simulink library "vmc"  (R2021b)
settings: Solver=VariableStepAuto  StartTime=0.0  StopTime=10.0  RelTol=1e-3
undefined symbols (not defined in the file or in its folder): AVMC_ACCDeltaTqIGain_X_kph, AVMC_ACCDeltaTqIGain_Y_mps2, AVMC_ACCDeltaTqPGain_X_kph, AVMC_ACCDeltaTqPGain_Y_kph, AVMC_ACCLongSteadyCtrl_X_kph, AVMC_AggressJerkPCT4AT_X_kph, AVMC_AggressJerkPCT_X_kph, AVMC_AggressLimitPCT4AT_X_kph, AVMC_AggressLimitPCT_X_kph, AVMC_CCLongSteadyCtrl_X_kph, AVMC_DISCDeltaTqIGain_X_kph, AVMC_DISCDeltaTqIGain_Y_mps2, AVMC_DISCDeltaTqPGain_X_kph, AVMC_DISCDeltaTqPGain_Y_kph, AVMC_DISCTrunAccJerk_X_s, AVMC_DISCTrunAccLimit_X_s, AVMC_ESCRegenOut_X_kph, AVMC_ESCRegenOut_Y_Deg, AVMC_ESCRegenOutEnSpd_X_Deg, AVMC_ISOAccLimit_X_mps, AVMC_ISODecLimit_X_mps, AVMC_ISOJerk_X_mps, AVMC_LatESCRegenOut_X_kph, AVMC_LatESCRegenOut_Y_Deg, AVMC_LongAccDeadZone_X_kph, AVMC_LongAccFiltTsforP2_X_Gps, AVMC_MCPresBaseTq_X_bar, AVMC_MSALongSteadyCtrl_X_kph, AVMC_MSAPedalOvrd2_X_kph, AVMC_MSAPedalOvrd_X_kph, AVMC_MSASpdBand_X_kph, AVMC_MSATqDownEndTq_X_kph, AVMC_MSATqDownTime_X_kph, AVMC_OPDDisSlideRate_X_Deg, AVMC_RDCDetectTime_X_kph, AVMC_RDCDetectTime_Y_pct, AVMC_RDCEnSlideRate_X_Deg, AVMC_RearWhlTqRatio_X_Nm, AVMC_RearWhlTqRatio_Y_gps, AVMC_RearWhlTqSlipGain_X_rat, AVMC_RearWhlTqSlipGain_Y_kph, AVMC_RearWhlTqSTRGGain_X_deg, AVMC_RearWhlTqSTRGGain_Y_kph, AVMC_RWSRrTSA2RWSPos_X_deg, AVMC_RWSSAS2FrtTSA_X_deg, AVMC_RWSVehSPD2RWSCoef_X_kph, AVMC_SoftJerkPCT_X_kph, AVMC_SoftLimitPCT_X_kph, AVMC_StESCYaw_X_kph, AVMC_StESCYaw_Y_Deg, AVMC_StESCYawCom_X_kph, AVMC_StESCYawCom_Y_Gps, AVMC_TMSpdBaseTq_X_rpm, AVMC_VehHoldBDecMap_X_kph, AVMC_VehHoldDecCtrlTime_X_kph, AVMC_VehHoldMCPPass_X_deg, C_TASK_10MS_S, C_TASK_5MS_S, DEG2RAD, ENUM_ACCAVAIL_AVAILABLE ... (+409)
libraries: hcu_lib x74, simulink x68, simulink_extras x3, $bdroot x2
(part 13 of 15)

== system vmc/VMC/VMC/Slide Rate  Calculation/4Wheel Calculation/RR Wheel ==
  VVMC_4WheelLongAcc_Gps : Inport
  task_time_s : Inport  Port=2
  VINP_RRRawWhlSpeed_kph : Inport  Port=3
  VTQD_GearActualPosn_enum : Inport  Port=4
  AND4 : Logic  Inputs=3  AllPortsSameDT=off  OutDataTypeStr=boolean
  Abs3 : Abs
  Add : Sum
  Add{3,8,15..16} (4 alike) : Sum  Inputs=+-
  Constant1 : Constant  Value=GRAVITY_G
  Constant11 : Constant  Value=KPH2MPS
  Constant14 : Constant  Value=ONE_PERCENT
  Constant15 : Constant  Value=KVMC_RawWhlSpeedDeadZone_kph
  Constant16 : Constant  Value=ZERO_FLOAT
  Constant17 : Constant  Value=KVMC_RawWhlSpeedDeadZone_kph
  Constant18 : Constant  Value=ONE_FLOAT
  Constant2 : Constant  Value=MPS2KPH
  Constant33 : Constant  Value=KPH2MPS
  Constant34 : Constant  Value=GRAVITY_G
  Constant35 : Constant  Value=KVMC_WhlSpdCalAccTs_c
  Constant42 : Constant  Value=KVMC_WheelSkidAccDev_Gps
  Constant43 : Constant  Value=KVMC_SkidRecVehSpdDev_kph
  Constant44 : Constant  Value=KPH2MPS
  Constant46 : Constant  Value=ENUM_GEARACTUALPOSN_D
  Constant47 : Constant  Value=ENUM_GEARACTUALPOSN_R
  Constant48 : Constant  Value=KVMC_PreVehSpdCalSW_flg
  Constant49 : Constant  Value=KVMC_RRWhlSkidReset_flg
  Constant5 : Constant  Value=KVMC_4WheelEnSkidDetSpd_kph
  Delay{,4..5,12..13,17} (6 alike) : Delay  DelayLength=1
  Divide3 : Product  Inputs=*//
  Divide7 : Product  Inputs=**//
  Equal : RelationalOperator  Operator===  OutDataTypeStr=boolean  RndMeth=Simplest
  Equal1 : RelationalOperator  Operator===  OutDataTypeStr=boolean  RndMeth=Simplest
  FirstOrderFilter3 : hcu_lib/Basic_Blocks/FirstOrderFilter
  OR : Logic  Operator=OR  AllPortsSameDT=off  OutDataTypeStr=boolean
  OR1 : Logic  Operator=OR  AllPortsSameDT=off  OutDataTypeStr=boolean
  OR2 : Logic  Operator=OR  AllPortsSameDT=off  OutDataTypeStr=boolean
  Product : Product
  Product1 : Product  Inputs=3
  Product2 : Product
  Product3 : Product
  Relational Operator14 : RelationalOperator  Operator=>  OutDataTypeStr=boolean  RndMeth=Simplest
  Relational Operator{2,5..6,15} (4 alike) : RelationalOperator  Operator=<=  OutDataTypeStr=boolean  RndMeth=Simplest
  SR_Latch3 : hcu_lib/Basic_Blocks/SR_Latch
  Saturation : Saturate  UpperLimit=KVMC_PredVehSpdLimit_mps  LowerLimit=ZERO_FLOAT
  Switch{,5..6,10} (4 alike) : Switch  Criteria=u2 > Threshold
  VVMC_RRPreVehSpd_kph : Outport
  VVMC_RRWhlSkid_flg : Outport  Port=2
  VVMC_RR4WhlSpdSlideRate_pct : Outport  Port=3
  wires:
  [VINP_RRRawWhlSpeed_kph] -> Add8/1
  Constant49/1 -> AND4/3
  Add8/1 -> Divide7/1
  [task_time_s] -> Divide7/3
  Add15/1 -> Abs3/1
  Relational Operator14/1 -> SR_Latch3/1
  [VVMC_4WheelLongAcc_Gps] -> Add16/2
  [task_time_s] -> FirstOrderFilter3/2
  [VINP_RRRawWhlSpeed_kph] -> Delay4/1
  Constant42/1 -> Relational Operator14/2
  FirstOrderFilter3/1 -> [VVMC_RRWhlCalAcc_Gps]  "VVMC_RRWhlCalAcc_Gps"
  Divide7/1 -> FirstOrderFilter3/1
  Relational Operator15/1 -> AND4/1
  Delay4/1 -> Add8/2
  Delay17/1 -> AND4/2
  [VVMC_RRWhlSkid_flg] -> Delay17/1
  Add16/1 -> Relational Operator14/1
  Delay12/1 -> Add15/1
  Constant43/1 -> Relational Operator15/2
  Delay13/1 -> Add15/2
  Constant33/1 -> Divide7/2
  Constant34/1 -> Divide7/4
  Abs3/1 -> Relational Operator15/1
  SR_Latch3/1 -> [VVMC_RRWhlSkid_flg]  "VVMC_RRWhlSkid_flg"
  [VVMC_RRWhlCalAcc_Gps] -> Add16/1
  Constant35/1 -> FirstOrderFilter3/3
  Constant14/1 -> Divide3/2
  Switch5/1 -> Divide3/3
  Divide3/1 -> Switch6/3  "VVMC_RRCal4WhlSpdSlideRate_pct"
  Switch6/1 -> [VVMC_RR4WhlSpdSlideRate_pct]  "VVMC_RR4WhlSpdSlideRate_pct"
  Constant18/1 -> Switch5/1
  Relational Operator6/1 -> Switch6/2
  [VINP_RRRawWhlSpeed_kph] -> Relational Operator6/1
  Relational Operator5/1 -> Switch5/2
  Constant15/1 -> Relational Operator6/2
  Constant16/1 -> Switch6/1
  Constant17/1 -> Relational Operator5/2
  [VINP_RRRawWhlSpeed_kph] -> Add3/1
  Add3/1 -> Divide3/1
  Product3/1 -> Switch/1
  Constant1/1 -> Product1/2
  Switch10/1 -> [VVMC_RRPreVehSpd_kph]  "VVMC_RRPreVehSpd_kph"
  [VINP_RRRawWhlSpeed_kph] -> Switch10/3
  [VTQD_GearActualPosn_enum] -> Equal/1
  Add/1 -> Product2/1  "VVMC_RRCalPreVehSpd_mps"
  Equal/1 -> OR/1
  Product2/1 -> Switch10/1
  [VVMC_4WheelLongAcc_Gps] -> Product1/1
  Constant11/1 -> Product/2
  Constant44/1 -> Product3/2
  [task_time_s] -> Product1/3
  Switch/1 -> Saturation/1  "VVMC_RRLastPreVehSpd_mps"
  [VVMC_RRPreVehSpd_kph] -> Delay5/1
  Delay/1 -> Product/1
  Constant47/1 -> Equal1/2
  Equal1/1 -> OR/2
  [VTQD_GearActualPosn_enum] -> Equal1/1
  Constant48/1 -> OR1/2
  Constant2/1 -> Product2/2
  OR1/1 -> Switch/2
  Constant46/1 -> Equal/2
  Product1/1 -> Add/1  "VVMC_RRDeltaVehSpd_mps"
  Saturation/1 -> Add/2
  Delay5/1 -> Product3/1
  Product/1 -> Switch/3
  OR/1 -> Switch10/2
  [VVMC_RRWhlSkid_flg] -> OR1/1
  [VINP_RRRawWhlSpeed_kph] -> Delay/1
  [VINP_RRRawWhlSpeed_kph] -> Delay13/1
  [VVMC_RRPreVehSpd_kph] -> Delay12/1
  [VVMC_RRPreVehSpd_kph] -> Add3/2
  [VVMC_RRPreVehSpd_kph] -> Relational Operator5/1
  [VVMC_RRPreVehSpd_kph] -> Switch5/3
  VVMC_4WheelLongAcc_Gps/1 -> [VVMC_4WheelLongAcc_Gps]
  VTQD_GearActualPosn_enum/1 -> [VTQD_GearActualPosn_enum]
  task_time_s/1 -> [task_time_s]
  VINP_RRRawWhlSpeed_kph/1 -> [VINP_RRRawWhlSpeed_kph]
  [VVMC_RRPreVehSpd_kph] -> VVMC_RRPreVehSpd_kph/1
  [VVMC_RRWhlSkid_flg] -> VVMC_RRWhlSkid_flg/1
  [VVMC_RR4WhlSpdSlideRate_pct] -> VVMC_RR4WhlSpdSlideRate_pct/1
  Constant5/1 -> Relational Operator2/2
  [VINP_RRRawWhlSpeed_kph] -> Relational Operator2/1
  Relational Operator2/1 -> OR2/1
  AND4/1 -> OR2/2
  OR2/1 -> SR_Latch3/2  "VVMC_RRWhlSkidReset_flg"

== system vmc/VMC/VMC/SafetyControl/Lateral_Module/Lateral_Reference_Model/Yaw_Rate_Difference_Equation ==
  note: I/O Area
  VINP_VehSpeed_kph : Inport
  VINP_SASAngle_deg : Inport  Port=2
  Constant2 : Constant  Value=KVMC_VehMass_kg
  ModelParameterCauculate : Subsystem
  Target Value Cauculate : Subsystem
  VVMC_TheoYawRateTS_degps : Outport
  wires:
  [VVMC_LatModelParaA12_enum] -> Target Value Cauculate/2(VVMC_LatModelParaA12_enum)
  [VVMC_LatModelParaA11_enum] -> Target Value Cauculate/1(VVMC_LatModelParaA11_enum)
  ModelParameterCauculate/4(VVMC_LatModelParaA22_enum) -> [VVMC_LatModelParaA22_enum]
  [VVMC_LatModelParaA21_enum] -> Target Value Cauculate/3(VVMC_LatModelParaA21_enum)
  ModelParameterCauculate/2(VVMC_LatModelParaA12_enum) -> [VVMC_LatModelParaA12_enum]
  Constant2/1 -> ModelParameterCauculate/1(KVMC_VehMass_kg)
  ModelParameterCauculate/1(VVMC_LatModelParaA11_enum) -> [VVMC_LatModelParaA11_enum]
  ModelParameterCauculate/3(VVMC_LatModelParaA21_enum) -> [VVMC_LatModelParaA21_enum]
  VINP_SASAngle_deg/1 -> [VINP_SASAngle_deg]
  VINP_VehSpeed_kph/1 -> [VINP_VehSpeed_kph]
  [VINP_VehSpeed_kph] -> ModelParameterCauculate/2(VINP_VehSpeed_kph)
  Target Value Cauculate/1(VVMC_TheoYawRateTS_degps) -> [VVMC_TheoYawRateTS_degps]
  [VVMC_TheoYawRateTS_degps] -> VVMC_TheoYawRateTS_degps/1
  ModelParameterCauculate/5(VVMC_LatModelParaB1_enum) -> [VVMC_LatModelParaB1_enum]
  ModelParameterCauculate/6(VVMC_LatModelParaB2_enum) -> [VVMC_LatModelParaB2_enum]
  [VVMC_LatModelParaA22_enum] -> Target Value Cauculate/4(VVMC_LatModelParaA22_enum)
  [VVMC_LatModelParaB1_enum] -> Target Value Cauculate/5(VVMC_LatModelParaB1_enum)
  [VVMC_LatModelParaB2_enum] -> Target Value Cauculate/6(VVMC_LatModelParaB2_enum)
  [VINP_SASAngle_deg] -> Target Value Cauculate/7(VINP_SASAngle_deg)

== system vmc/VMC/VMC/SafetyControl/Lateral_Module/Lateral_Reference_Model/Yaw_Rate_Steady_State_Equaltion ==
  note: Steady-State Yaw Rate equaltion:
      | Yaw Rate = (V*SWA*g*57.3)/(57.3*L*g+KV.^2)
  VINP_VehSpeed_kph : Inport
  VINP_SASAngle_deg : Inport  Port=2
  (m) : Constant  Value=KVMC_WheelBase_m
  Add : Sum
  Data Type Conversion : DataTypeConversion  OutDataTypeStr=single
  Divide : Product  Inputs=*/
  Product{,1..7} (8 alike) : Product
  Square : Math  Operator=square  SaturateOnIntegerOverflow=on
  const : Constant  Value=KPH2MPS  SampleTime=-1
  const1 : Constant  Value=KVMC_SWAGR_rat  SampleTime=-1
  const2 : Constant  Value=RAD2DEG  SampleTime=-1
  const3 : Constant  Value=GRAVITY_G  SampleTime=-1
  const4 : Constant  Value=KVMC_USGradient_enum  SampleTime=-1
  const5 : Constant  Value=RAD2DEG  SampleTime=-1
  const6 : Constant  Value=GRAVITY_G  SampleTime=-1
  VVMC_TheoYawRateSS_degps : Outport
  wires:
  Product1/1 -> Divide/1
  Product2/1 -> Add/1
  Add/1 -> Divide/2
  Product5/1 -> Product1/1
  Product/1 -> Product4/1, Square/1
  Product4/1 -> Product5/1
  Product3/1 -> Product1/2
  Square/1 -> Product2/1
  Product7/1 -> Add/2
  Divide/1 -> Data Type Conversion/1
  const4/1 -> Product2/2
  VINP_SASAngle_deg/1 -> Product3/1
  VINP_VehSpeed_kph/1 -> Product/1
  Data Type Conversion/1 -> VVMC_TheoYawRateSS_degps/1
  const/1 -> Product/2
  const1/1 -> Product3/2
  const2/1 -> Product4/2
  const3/1 -> Product5/2
  (m)/1 -> Product6/1
  const5/1 -> Product6/2
  Product6/1 -> Product7/1
  const6/1 -> Product7/2

== system vmc/VMC/VMC/SafetyControl/Lateral_Module/Lateral_Reference_Model/Yaw_Rate_Difference_Equation/ModelParameterCauculate ==
  KVMC_VehMass_kg : Inport
  VINP_VehSpeed_kph : Inport  Port=2
  Add : Sum
  Add1 : Sum
  Add2 : Sum  Inputs=+-
  Add3 : Sum
  Constant{1,13,17,21..22} (5 alike) : Constant  Value=KVMC_CorStiffF_enum  SampleTime=-1
  Constant10 : Constant  Value=KVMC_Izz_kgpm2  SampleTime=-1
  Constant15 : Constant  Value=KVMC_CorStiffR_enum  SampleTime=-1
  Constant18 : Constant  Value=KVMC_CorStiffR_enum  SampleTime=-1
  Constant19 : Constant  Value=KVMC_Lengthb_m  SampleTime=-1
  Constant2 : Constant  Value=KVMC_CorStiffR_enum  SampleTime=-1
  Constant20 : Constant  Value=KVMC_Lengtha_m  SampleTime=-1
  Constant23 : Constant  Value=KVMC_Lengtha_m  SampleTime=-1
  Constant24 : Constant  Value=KVMC_Izz_kgpm2  SampleTime=-1
  Constant3 : Constant  Value=KVMC_Lengtha_m  SampleTime=-1
  Constant4 : Constant  Value=KVMC_Lengthb_m  SampleTime=-1
  Constant5 : Constant  Value=MINUSONE_FLOAT  SampleTime=-1
  Constant6 : Constant  Value=KPH2MPS  SampleTime=-1
  Constant7 : Constant  Value=MINUSONE_FLOAT  SampleTime=-1
  Constant8 : Constant  Value=MINUSONE_FLOAT  SampleTime=-1
  Divide{,1..2,4..5} (5 alike) : Product  Inputs=*/
  Divide3 : Product  Inputs=/*
  Product{,1..10} (11 alike) : Product
  Saturation : Saturate  UpperLimit=inf  LowerLimit=10
  Square : Math  Operator=square  SaturateOnIntegerOverflow=on
  Square1 : Math  Operator=square  SaturateOnIntegerOverflow=on
  VVMC_LatModelParaA11_enum : Outport
  VVMC_LatModelParaA12_enum : Outport  Port=2
  VVMC_LatModelParaA21_enum : Outport  Port=3
  VVMC_LatModelParaA22_enum : Outport  Port=4
  VVMC_LatModelParaB1_enum : Outport  Port=5
  VVMC_LatModelParaB2_enum : Outport  Port=6
  wires:
  Add2/1 -> VVMC_LatModelParaA12_enum/1  "(-cf *a+cr *b) / (M*vx) - Vx"
  Constant21/1 -> Divide4/1
  [VVMC_Paras2_enum] -> Divide1/1
  Constant6/1 -> Product1/2
  Product8/1 -> Divide/1  "-(cf+cr)"
  Product2/1 -> Add3/1  "a^2 *cf"
  Constant18/1 -> Product3/2
  Constant10/1 -> Product5/2
  Constant3/1 -> Product6/2  "a"
  [VVMC_VehSpeed_mps] -> Product9/2
  Constant23/1 -> Product4/2
  KVMC_VehMass_kg/1 -> [KVMC_VehMass_kg]
  Constant1/1 -> Add/1
  Add1/1 -> [VVMC_Paras2_enum]  "-cf *a + cr *b"
  Add3/1 -> Product10/1
  Product1/1 -> [VVMC_VehSpeed_mps]  "Vx"
  Constant4/1 -> Product/2  "b"
  Constant13/1 -> Product7/1
  Divide2/1 -> VVMC_LatModelParaA21_enum/1  "(-cf *a+cr *b) / (Izz *Vx)"
  Divide1/1 -> Add2/1  "(-cf *a+cr *b) / (M*vx)"
  Product9/1 -> [VVMC_Paras1_enum]  "M*Vx"
  [VVMC_Paras1_enum] -> Divide/2
  Product4/1 -> Divide5/1
  [VVMC_Paras1_enum] -> Divide1/2
  [KVMC_VehMass_kg] -> Product9/1
  [VVMC_Paras2_enum] -> Divide2/1
  Divide/1 -> VVMC_LatModelParaA11_enum/1  "-(cf+cr)/(M*Vx)"
  Square1/1 -> Product3/1  "b^2"
  Constant15/1 -> Product/1
  Product6/1 -> Add1/1  "-cf *a"
  Constant2/1 -> Add/2
  Product/1 -> Add1/2  "cr *b"
  Divide4/1 -> VVMC_LatModelParaB1_enum/1  "Cf/M"
  VINP_VehSpeed_kph/1 -> [VINP_VehSpeed_kph]
  [KVMC_VehMass_kg] -> Divide4/2
  Divide3/1 -> VVMC_LatModelParaA22_enum/1  "-(cf*a^2+cr*b^2) / (Izz *Vx)"
  Saturation/1 -> Product1/1
  [VINP_VehSpeed_kph] -> Saturation/1
  Divide5/1 -> VVMC_LatModelParaB2_enum/1  "Cf*a/Izz"
  Product3/1 -> Add3/2  "b^2 *cr"
  Add/1 -> Product8/1
  [VVMC_VehSpeed_mps] -> Product5/1
  [VVMC_Paras3_enum] -> Divide2/2
  Constant22/1 -> Product4/1
  [VVMC_Paras3_enum] -> Divide3/1
  Constant17/1 -> Product2/2
  [VVMC_VehSpeed_mps] -> Add2/2
  Product5/1 -> [VVMC_Paras3_enum]  "Izz *Vx"
  Constant24/1 -> Divide5/2
  Square/1 -> Product2/1  "a^2"
  Constant20/1 -> Square/1  "a"
  Constant19/1 -> Square1/1  "b"
  Constant5/1 -> Product7/2
  Product7/1 -> Product6/1
  Constant7/1 -> Product8/2
  Constant8/1 -> Product10/2
  Product10/1 -> Divide3/2

== system vmc/VMC/VMC/SafetyControl/Lateral_Module/Lateral_Reference_Model/Yaw_Rate_Difference_Equation/Target Value Cauculate ==
  note: I/O Area
  VVMC_LatModelParaA11_enum : Inport
  VVMC_LatModelParaA12_enum : Inport  Port=2
  VVMC_LatModelParaA21_enum : Inport  Port=3
  VVMC_LatModelParaA22_enum : Inport  Port=4
  VVMC_LatModelParaB1_enum : Inport  Port=5
  VVMC_LatModelParaB2_enum : Inport  Port=6
  VINP_SASAngle_deg : Inport  Port=7
  Add4 : Sum  Inputs=+++
  Add5 : Sum
  Add6 : Sum
  Add7 : Sum  Inputs=+++
  Constant : Constant  Value=MPS2KPH  SampleTime=-1
  Constant{1..2,7,9..10} (5 alike) : Constant  Value=C_TASK_10MS_S  SampleTime=-1
  Constant3 : Constant  Value=RAD2DEG  SampleTime=-1
  Constant4 : Constant  Value=KVMC_SWAGR_rat  SampleTime=-1
  Constant5 : Constant  Value=DEG2RAD  SampleTime=-1
  Constant6 : Constant  Value=ONE_FLOAT  SampleTime=-1
  Constant8 : Constant  Value=ONE_FLOAT  SampleTime=-1
  Data Type Conversion : DataTypeConversion  OutDataTypeStr=single
  Data Type Conversion1 : DataTypeConversion  OutDataTypeStr=single
  Delay{,1..4} (5 alike) : Delay  DelayLength=1
  Product{,1..14} (15 alike) : Product
  VVMC_TheoYawRateTS_degps : Outport
  wires:
  [YawRate_desired_rad_s] -> Delay1/1
  Constant10/1 -> Product13/2
  Constant3/1 -> Product3/2
  Product2/1 -> Product8/1
  VVMC_LatModelParaB2_enum/1 -> [VVMC_LatModelParaB2_enum]
  [VVMC_LatModelParaB1_enum] -> Product11/2
  Constant5/1 -> Product9/2
  Product10/1 -> Data Type Conversion/1  "dt*SWA(K-1)"
  Constant7/1 -> Product10/2
  [P1] -> Product14/1
  [VVMC_LatModelParaB2_enum] -> Product14/2
  Data Type Conversion/1 -> [P1]
  [Vy_d_Mps] -> Delay/1
  [P1] -> Product11/1
  [VVMC_LatModelParaA12_enum] -> Product2/1
  VVMC_LatModelParaA11_enum/1 -> [VVMC_LatModelParaA11_enum]
  Product5/1 -> Add4/2
  Product11/1 -> Add7/3  "b1*dt*SWA(K-1)"
  VVMC_LatModelParaA22_enum/1 -> [VVMC_LatModelParaA22_enum]
  Constant4/1 -> Product6/2
  Delay3/1 -> Product7/2  "Vy_d(K-1)"
  VVMC_LatModelParaB1_enum/1 -> [VVMC_LatModelParaB1_enum]
  [YawRate_desired_rad_s] -> Delay4/1
  VVMC_LatModelParaA21_enum/1 -> [VVMC_LatModelParaA21_enum]
  Delay4/1 -> Product8/2  "YawRate_d(K-1)"
  Constant9/1 -> Product12/2
  [YawRate_desired_rad_s] -> Product3/1
  Add7/1 -> [Vy_d_Mps]  "Vy_d(Mps)"
  [Vy_d_Mps] -> Product/1
  Constant2/1 -> Product2/2
  VINP_SASAngle_deg/1 -> [VINP_SASAngle_deg]
  Product12/1 -> Product4/2
  Product1/1 -> Add6/1
  VVMC_LatModelParaA12_enum/1 -> [VVMC_LatModelParaA12_enum]
  [VINP_SASAngle_deg] -> Product6/1
  Product9/1 -> Delay2/1
  Product8/1 -> Add7/2  "a12*dt*YawRate_d(K-1)"
  Product4/1 -> Add4/1  "a21*dt*Vy_d(K-1)"
  Add5/1 -> Product5/1
  Product6/1 -> Product9/1
  Constant6/1 -> Add5/1
  Constant1/1 -> Product1/2
  Delay1/1 -> Product5/2  "YawRate_d(K-1)"
  [VVMC_LatModelParaA22_enum] -> Product13/1
  Add6/1 -> Product7/1
  Product7/1 -> Add7/1  "(1+a11*dt)*Vy_d(K-1)"
  Constant8/1 -> Add6/2
  [Vy_d_Mps] -> Delay3/1
  Constant/1 -> Product/2
  Product13/1 -> Add5/2
  Delay/1 -> Product4/1  "Vy_d(K-1)"
  Delay2/1 -> Product10/1
  Product14/1 -> Add4/3  "b2*dt*SWA(K-1)"
  [VVMC_LatModelParaA21_enum] -> Product12/1
  Product3/1 -> Data Type Conversion1/1  "YawRate_desired(deg/s)"
  Add4/1 -> [YawRate_desired_rad_s]  "YawRate_desired(rad/s)"
  [VVMC_LatModelParaA11_enum] -> Product1/1
  Data Type Conversion1/1 -> [VVMC_TheoYawRateTS_degps]
  [VVMC_TheoYawRateTS_degps] -> VVMC_TheoYawRateTS_degps/1
  Product/1 -> [VVMC_VyDesired_kph]  "VVMC_VyDesired_kph"

== stateflow chart vmc/VMC/VMC/SPD2ACC/SPD2ACC Active Determination/SPD2ACC Active Determination ==
  state SPD2ACCActiveDetermination
    (default) -> (junction 4) : {VVMC_SPD2ACCAct_flg = FALSE}
    SPD2ACCActiveDetermination -> (junction 4)
    (junction 4) -> (junction 7) [order 1] : [VVMC_FeatArbitrSta_enum == ENUM_FEATARBITRSTA_DISC ||...
        |  VVMC_FeatArbitrSta_enum == ENUM_FEATARBITRSTA_CC ||...
        |  VVMC_FeatArbitrSta_enum == ENUM_FEATARBITRSTA_MSA ||...
        |  VVMC_FeatArbitrSta_enum == ENUM_FEATARBITRSTA_ACCDISC]
    (junction 4) -> (junction 12) [order 2] : {VVMC_SPD2ACCAct_flg = FALSE}
    (junction 7) -> (junction 10) : {VVMC_SPD2ACCAct_flg = TURE}
  data: VVMC_FeatArbitrSta_enum input uint8; VVMC_SPD2ACCAct_flg output boolean; TURE input boolean; FALSE input boolean; ENUM_FEATARBITRSTA_DISC input uint8; ENUM_FEATARBITRSTA_ACCDISC input uint8; ENUM_FEATARBITRSTA_CC input; ENUM_FEATARBITRSTA_MSA input

== stateflow chart vmc/VMC/VMC/MSA function/MSAActivationHandshake/Chart ==
  state MSA_Handshaking
    (default) -> (junction 391) : {VVMC_MSACtrlSta_enum = 0;
        |  VVMC_MSASpdWar_flg = 0;
        |  VVMC_WaitResetSpdLoop_flg = 0;}
    MSA_Handshaking -> (junction 391) [order 4] : {VVMC_WaitResetSpdLoop_flg = 0;
        |  VVMC_CheckMeterSpdLoop_flg = 0;
        |  VVMC_CheckCmdLoop_flg = 0}
    (junction 391) -> (junction 463) [order 1] : [VTQD_SpdCtrlMode_enum == 3 ||...
        | VTQD_SpdCtrlMode_enum == 4]
        | %add20230706
    (junction 463) -> (junction 392) [order 1] : [VTQD_ExternalTqAllow_flg]
    (junction 391) -> (junction 467) [order 2] : {VVMC_MSACtrlSta_enum = 0;}
        | %Phase2 VVMC_MSAActive_flg = 0;}
        | %add20230706
    (junction 463) -> (junction 468) [order 2] : {VVMC_MSACtrlSta_enum = 5;}
        | %Phase2  VVMC_MSAActive_flg = 0;}
        | %add20230706
    (junction 392) -> (junction 389) : {VVMC_MSACtrlSta_enum = 1;}
    MSA_Handshaking -> (junction 389) [order 3] : [VVMC_WaitResetSpdLoop_flg && VTQD_ExternalTqAllow_flg]
        | {VVMC_WaitResetSpdLoop_flg = 0;} %add20230705
    (junction 389) -> (junction 464) [order 1] : [VVMC_FeatSetSpdForCalcu_kph > ONE_FLOAT]
    (junction 389) -> (junction 469) [order 2]
    (junction 464) -> (junction 330)
    MSA_Handshaking -> (junction 330) [order 1] : [VVMC_CheckMeterSpdLoop_flg && VTQD_ExternalTqAllow_flg]
        | {VVMC_CheckMeterSpdLoop_flg = 0;}
        | %Phase2 add
    (junction 330) -> (junction 332) [order 1] : [VVMC_FeatSetSpdForCalcu_kph >= KVMC_MSAActiveMetSpdLo_kph &&...
        |  VVMC_FeatSetSpdForCalcu_kph <=  KVMC_MSAActiveMetSpdHi_kph]
    (junction 330) -> (junction 338) [order 2] : {VVMC_MSASpdWar_flg = 0;}
    (junction 332) -> (junction 335) : {VVMC_MSACtrlSta_enum = 2;}
        | %Phase2 VVMC_MSAActive_flg = 1;}
    (junction 338) -> (junction 339) [order 1] : [VVMC_FeatSetSpdForCalcu_kph > KVMC_MSAActiveMetSpdHi_kph]
    (junction 335) -> (junction 336) [order 1] : [(VVMC_MeterIndSpeedForCalcu_kph - VVMC_FeatSetSpdForCalcu_kph)...
        | >= KVMC_CCMSASpdWar_kph]
    (junction 338) -> (junction 334) [order 2] : {VVMC_MSACtrlSta_enum = 3;}
    (junction 339) -> (junction 333) : {VVMC_MSACtrlSta_enum = 4;}
    (junction 335) -> (junction 346) [order 2] : {VVMC_MSASpdWar_flg = 0;}
    (junction 336) -> (junction 345) : {VVMC_MSASpdWar_flg = 1;}
    (junction 334) -> (junction 333)
    (junction 333) -> (junction 337) : {VVMC_WaitResetSpdLoop_flg = 1;}
    (junction 346) -> (junction 345)
    (junction 345) -> (junction 342) [order 1] : [(VTQD_SpdCtrlMode_enum != 3 && VTQD_SpdCtrlMode_enum != 4) ||...
        |   VVMC_DetectSWCCANCEL_flg == 1||...
        |  !VTQD_ExternalTqAllow_flg] %Phase2 add20230815
        | %add20230706
    (junction 345) -> (junction 471) [order 2]
    (junction 342) -> (junction 348) : {VVMC_MSASpdWar_flg = 0;}
    (junction 471) -> (junction 472) [order 1] : [VVMC_MSAOvrdAllow_flg == 1]
    (junction 471) -> (junction 474) [order 2] : {VVMC_MSACtrlSta_enum = 2;}
    (junction 472) -> (junction 473) : {VVMC_MSACtrlSta_enum = 7;}
    (junction 474) -> (junction 473)
    (junction 473) -> (junction 347) : {VVMC_CheckMeterSpdLoop_flg = 1;}
    (junction 348) -> (junction 343) [order 1] : [!VTQD_ExternalTqAllow_flg] %Phase2 add20230815
    (junction 348) -> (junction 360) [order 2]
    (junction 343) -> (junction 344) : %Phase2 add20230815
        | {VVMC_MSACtrlSta_enum = 5;}
        | %Back to outer first loop.
    MSA_Handshaking -> (junction 360) [order 2] : [VVMC_CheckCmdLoop_flg && VTQD_ExternalTqAllow_flg]
        | {VVMC_CheckCmdLoop_flg = 0;} %Phase2 add 20231003
    (junction 360) -> (junction 350) [order 1] : [(VTQD_SpdCtrlMode_enum != 3 && VTQD_SpdCtrlMode_enum != 4)] %Phase2 add
    (junction 360) -> (junction 353) [order 2] : %Phase2 {VVMC_MSAActive_flg = 0;
        | {VVMC_MSACtrlSta_enum = 1;}
    (junction 350) -> (junction 373) : %Phase2 {VVMC_MSAActive_flg = 0;
        | {VVMC_MSACtrlSta_enum = 0;}
        |  %Back to outer first loop.
    (junction 353) -> (junction 354) [order 1] : [VVMC_DetectSWCRes_flg == 1 ||...
        |  VVMC_DetectSWCSet_flg == 1]
        | %Phase2 add
    (junction 353) -> (junction 370) [order 2] : {VVMC_CheckCmdLoop_flg = 1}
        | %Phase2 Modify 20231003
    (junction 354) -> (junction 349) : {VVMC_WaitResetSpdLoop_flg = 1}
        | %Phase2 add
  data: VTQD_SpdCtrlMode_enum input uint8; VVMC_MSACtrlSta_enum output uint8; VVMC_MSASpdWar_flg output boolean; VTQD_ExternalTqAllow_flg input boolean; KVMC_MSAActiveMetSpdHi_kph input single; VVMC_MeterIndSpeedForCalcu_kph input single; KVMC_MSAActiveMetSpdLo_kph input single; VVMC_FeatSetSpdForCalcu_kph input single; KVMC_CCMSASpdWar_kph input single; VVMC_DetectSWCCANCEL_flg input boolean; VVMC_MSAOvrdAllow_flg input; VVMC_CheckMeterSpdLoop_flg local boolean; VVMC_WaitResetSpdLoop_flg local boolean; VVMC_DetectSWCRes_flg input boolean; VVMC_DetectSWCSet_flg input boolean; VVMC_CheckCmdLoop_flg local boolean; ONE_FLOAT parameter

== stateflow chart vmc/VMC/VMC/CruiseControlFunction/CCActiveDetermination/Chart ==
  state CCActiveDetermination
    (default) -> (junction 360) : {
        |  VVMC_CCCtrlSta_enum = 0;
        |  VVMC_CCSpdWar_flg = 0;
        |  VVMC_SWCResUpLoop_flg = 0;
        |  VVMC_CruzLoopSpdChk_flg = 0;
        |  VVMC_CheckCmdLoop_flg = 0;
        |  }
    CCActiveDetermination -> (junction 360) [order 4] : {VVMC_SWCResUpLoop_flg = 0;
        |  VVMC_CheckCmdLoop_flg = 0;
        |  VVMC_CruzLoopSpdChk_flg = 0;}
    (junction 360) -> (junction 353) [order 1] : [VTQD_SpdCtrlMode_enum == 2]
    (junction 353) -> (junction 347) [order 1] : [VTQD_ExternalTqAllow_flg]
    (junction 360) -> (junction 343) [order 2] : {VVMC_CCCtrlSta_enum = 0;}
        | %Phase2 VVMC_CruzActive_flg = 0;}
        | %Back to first loop
        | %add20230706
    (junction 353) -> (junction 367) [order 2] : {VVMC_CCCtrlSta_enum = 5;}
        | %Phase2 VVMC_CruzActive_flg = 0;}
        | %Back to first loop
        | %add20230706
    (junction 347) -> (junction 361) : {VVMC_CCCtrlSta_enum = 1;}
    CCActiveDetermination -> (junction 361) [order 3] : [VVMC_SWCResUpLoop_flg && VTQD_ExternalTqAllow_flg]{VVMC_SWCResUpLoop_flg = 0;} %add20230705 %Phase2 modify
    (junction 361) -> (junction 368) [order 1] : [VVMC_FeatSetSpdForCalcu_kph > ONE_FLOAT &&...
        |  VINP_ADASAEBSta_enum ~= ENUM_ADASAEBSTA_ACTIVE]
    (junction 361) -> (junction 374) [order 2] : %Back to first loop
    (junction 368) -> (junction 344)
    CCActiveDetermination -> (junction 344) [order 1] : [VVMC_CruzLoopSpdChk_flg && VTQD_ExternalTqAllow_flg]{VVMC_CruzLoopSpdChk_flg = 0;} %add20230705
    (junction 344) -> (junction 345) [order 1] : [VVMC_FeatSetSpdForCalcu_kph >= KVMC_CCActiveMetSpdLo_kph &&...
        |  VVMC_FeatSetSpdForCalcu_kph <= KVMC_CCActiveMetSpdHi_kph]
    (junction 344) -> (junction 370) [order 2] : {VVMC_CCSpdWar_flg = 0;}
    (junction 345) -> (junction 375) : %Phase 2 {VVMC_CruzActive_flg = 1;
        | {VVMC_CCCtrlSta_enum = 2;}
    (junction 370) -> (junction 371) [order 1] : [VVMC_FeatSetSpdForCalcu_kph < KVMC_CCActiveMetSpdLo_kph]
    (junction 370) -> (junction 348) [order 2] : {VVMC_CCCtrlSta_enum = 4;}
        | %TBD
    (junction 371) -> (junction 346) : {VVMC_CCCtrlSta_enum = 3;}
        | %TBD
    (junction 346) -> (junction 348)
    (junction 348) -> (junction 355) : {VVMC_SWCResUpLoop_flg = 1;}
    (junction 375) -> (junction 349) [order 1] : [(VINP_VehSpeed_kph - VVMC_FeatSetSpdForCalcu_kph) >=...
        |  KVMC_CCMSASpdWar_kph]
    (junction 375) -> (junction 356) [order 2] : {VVMC_CCSpdWar_flg = 0;}
    (junction 349) -> (junction 363) : {VVMC_CCSpdWar_flg = 1;}
    (junction 363) -> (junction 356)
    (junction 356) -> (junction 376)
    (junction 376) -> (junction 350) [order 1] : [VVMC_CCPedalOvrd_flg]
    (junction 376) -> (junction 351) [order 2] : {VVMC_CCCtrlSta_enum = 2}
    (junction 350) -> (junction 358) : {VVMC_CCCtrlSta_enum = 7}
    (junction 358) -> (junction 351)
    (junction 351) -> (junction 352)
    (junction 352) -> (junction 354) [order 1] : [ VTQD_SpdCtrlMode_enum != 2 ||...
        |   VVMC_DetectSWCCANCEL_flg ||...
        |   VINP_BrkSwSta_flg ||...
        |   VINP_BrakeSWGPIO_flg  ||...
        |   VINP_ADASAEBSta_enum == ENUM_ADASAEBSTA_ACTIVE] %Phase2 add
    (junction 352) -> (junction 357) [order 2] : {VVMC_CruzLoopSpdChk_flg = 1;}
        | %Phase2 modify
    (junction 354) -> (junction 359) : {VVMC_CCSpdWar_flg = 0;}
    CCActiveDetermination -> (junction 359) [order 2] : [VVMC_CheckCmdLoop_flg && VTQD_ExternalTqAllow_flg]{VVMC_CheckCmdLoop_flg = 0;}
    (junction 359) -> (junction 362) [order 1] : [VTQD_SpdCtrlMode_enum == 2]
    (junction 359) -> (junction 364) [order 2] : %Phase2 {VVMC_CruzActive_flg = 0;
        | {VVMC_CCCtrlSta_enum = 0;}
        | %Back to first loop
    (junction 362) -> (junction 365) : %Phase 2 {VVMC_CruzActive_flg = 0;
        | {VVMC_CCCtrlSta_enum = 1;
        |  VVMC_SWCSetDownLoop_flg = 1;} %Phase2 add
    (junction 365) -> (junction 432) [order 1] : [VVMC_DetectSWCResUp_flg == 1 ||...
        |  VVMC_DetectSWCSetDown_flg == 1]
        | %Phase2 add
    (junction 365) -> (junction 431) [order 2] : {VVMC_CheckCmdLoop_flg = 1}
    (junction 432) -> (junction 433) : {VVMC_SWCResUpLoop_flg = 1}
        | %Phase2 add
  CCActiveDetermination -> CCActiveDetermination [order 1] : [!VTQD_ExternalTqAllow_flg || VTQD_GearActualPosn_enum ~= ENUM_GEARACTUALPOSN_D]
      | %add20231101
  data: VVMC_CCCtrlSta_enum output uint8; VTQD_SpdCtrlMode_enum input uint8; VVMC_CCSpdWar_flg output boolean; VTQD_ExternalTqAllow_flg input boolean; VVMC_DetectSWCSetDown_flg input boolean; KVMC_CCActiveMetSpdHi_kph input single; VINP_VehSpeed_kph input single; KVMC_CCActiveMetSpdLo_kph input single; VVMC_FeatSetSpdForCalcu_kph input single; KVMC_CCMSASpdWar_kph input single; VINP_BrakeSWGPIO_flg input boolean; VVMC_DetectSWCCANCEL_flg input boolean; VINP_BrkSwSta_flg input boolean; VVMC_DetectSWCResUp_flg input boolean; VVMC_CruzLoopSpdChk_flg local boolean; VVMC_SWCSetDownLoop_flg local boolean; VINP_ADASAEBSta_enum input uint8; ENUM_ADASAEBSTA_ACTIVE input uint8; VVMC_CCPedalOvrd_flg input boolean; VTQD_GearActualPosn_enum input uint8; ENUM_GEARACTUALPOSN_D input uint8; VVMC_CheckCmdLoop_flg local boolean; VVMC_SWCResUpLoop_flg local boolean; ONE_FLOAT parameter

== stateflow chart vmc/VMC/VMC/ACC_Function/ACC Torque Source Determination/TimeGapJudgement ==
  state TimeGapJudgement
    (default) -> (junction 11) : {VVMC_TimeGapJudge_flag = FALSE}
    TimeGapJudgement -> (junction 11)
    (junction 11) -> (junction 71) [order 1] : [(VINP_VehSpeed_kph * KPH2MPS - VINP_ACCObjRelSpd_mps) > ZERO_FLOAT]
    (junction 11) -> (junction 33) [order 2] : {VVMC_TimeGapJudge_flag = FALSE;
        |  VVMC_TimeGapCalcu_s = KVMC_TimeGapMax_s}
    (junction 71) -> (junction 24) : {VVMC_TimeGapCalcu_s = VINP_ACCObjDist_m / (VINP_VehSpeed_kph * KPH2MPS - VINP_ACCObjRelSpd_mps)}
    (junction 24) -> (junction 29) [order 1] : [VINP_TimeGapLevel_enum == ENUM_TIMEGAPLEVEL_LEVEL1]
    (junction 29) -> (junction 27) [order 1] : [VVMC_TimeGapCalcu_s <= KVMC_TimeGapBandLv1_s]
    (junction 24) -> (junction 35) [order 2]
    (junction 29) -> (junction 44) [order 2] : {VVMC_TimeGapJudge_flag = FALSE}
    (junction 27) -> (junction 31) : {VVMC_TimeGapJudge_flag = TRUE}
    (junction 35) -> (junction 38) [order 1] : [VINP_TimeGapLevel_enum == ENUM_TIMEGAPLEVEL_LEVEL2]
    (junction 38) -> (junction 42) [order 1] : [VVMC_TimeGapCalcu_s <= KVMC_TimeGapBandLv2_s]
    (junction 35) -> (junction 56) [order 2]
    (junction 38) -> (junction 46) [order 2] : {VVMC_TimeGapJudge_flag = FALSE}
    (junction 42) -> (junction 40) : {VVMC_TimeGapJudge_flag = TRUE}
    (junction 56) -> (junction 49) [order 1] : [VINP_TimeGapLevel_enum == ENUM_TIMEGAPLEVEL_LEVEL3]
    (junction 49) -> (junction 50) [order 1] : [VVMC_TimeGapCalcu_s <= KVMC_TimeGapBandLv3_s]
    (junction 56) -> (junction 59) [order 2]
    (junction 49) -> (junction 48) [order 2] : {VVMC_TimeGapJudge_flag = FALSE}
    (junction 50) -> (junction 53) : {VVMC_TimeGapJudge_flag = TRUE}
    (junction 59) -> (junction 65) [order 1] : [VINP_TimeGapLevel_enum == ENUM_TIMEGAPLEVEL_LEVEL4]
    (junction 65) -> (junction 64) [order 1] : [VVMC_TimeGapCalcu_s <= KVMC_TimeGapBandLv4_s]
    (junction 59) -> (junction 68) [order 2] : {VVMC_TimeGapJudge_flag = FALSE}
    (junction 65) -> (junction 66) [order 2] : {VVMC_TimeGapJudge_flag = FALSE}
    (junction 64) -> (junction 58) : {VVMC_TimeGapJudge_flag = TRUE}
  data: VINP_ACCObjRelSpd_mps input; VINP_ACCObjDist_m input single; VINP_VehSpeed_kph input single; KPH2MPS input single; VINP_TimeGapLevel_enum input uint8; VVMC_TimeGapJudge_flag output boolean; ENUM_TIMEGAPLEVEL_LEVEL1 input uint8; KVMC_TimeGapBandLv1_s input single; ENUM_TIMEGAPLEVEL_LEVEL2 input uint8; KVMC_TimeGapBandLv2_s input single; ENUM_TIMEGAPLEVEL_LEVEL3 input uint8; KVMC_TimeGapBandLv3_s input single; ENUM_TIMEGAPLEVEL_LEVEL4 input uint8; KVMC_TimeGapBandLv4_s input single; TRUE input boolean; FALSE input boolean; ZERO_FLOAT input single; KVMC_TimeGapMax_s input single; VVMC_TimeGapCalcu_s output single

== stateflow chart vmc/VMC/VMC/SPD2ACC/ReqACCCalcu/CMDRepeat ==
  state CMDCycleTime
    (default) -> (junction 4) : {VVMC_CMDCount_enum = ZERO_INT}
    CMDCycleTime -> (junction 4)
    (junction 4) -> (junction 8) [order 1] : [VVMC_SPD2ACCAct_flg == TRUE &&...
        | (VVMC_ReqAccCalcu_mps2 > ZERO_FLOAT ||...
        |  VVMC_ReqAccCalcu_mps2 < ZERO_FLOAT) &&...
        |  VVMC_AbsDeltaSpd_kph > ZERO_FLOAT]
    (junction 8) -> (junction 13) [order 1] : [VVMC_CMDCount_enum == ZERO_INT]
    (junction 4) -> (junction 21) [order 2] : {VVMC_ReqAcc_mps2 = ZERO_FLOAT;
        |  VVMC_CMDCount_enum = ZERO_INT}
    (junction 8) -> (junction 11) [order 2]
    (junction 13) -> (junction 15) : {VVMC_ReqAcc_mps2 = VVMC_ReqAccCalcu_mps2;
        |  VVMC_CMDCount_enum++}
    (junction 11) -> (junction 17) [order 1] : [VVMC_CMDCount_enum < KVMC_CMDRepeatTime_enum]
    (junction 11) -> (junction 23) [order 2] : {VVMC_CMDCount_enum = ZERO_INT}
    (junction 17) -> (junction 19) : {VVMC_CMDCount_enum++}
  data: VVMC_AbsDeltaSpd_kph input; VVMC_ReqAccCalcu_mps2 input single; TRUE input; ZERO_FLOAT input; VVMC_CMDCount_enum local uint8; VVMC_ReqAcc_mps2 output single; ZERO_INT input uint8; KVMC_CMDRepeatTime_enum input uint8; VVMC_SPD2ACCAct_flg input

== stateflow chart vmc/VMC/VMC/SPD2ACC/ReqACCCalcu/ConstantSpeedControl1 ==
  state ConstantSpeedControl
    (default) -> (junction 2) : {SpdCtrlFlag = 0;
        |  ReqAccel = 0}
    ConstantSpeedControl -> (junction 2)
    (junction 2) -> (junction 6) [order 1] : [DeltaSpeed >= KVMC_SpdCtrlEnBand_kph && SpdCtrlFlag == 0]
    (junction 2) -> (junction 16) [order 2]
    (junction 6) -> (junction 8) : {SpdCtrlFlag = 1;
        |  ReqAccel = MINUSONE_FLOAT * KVMC_SpdCtrlReqAccel_mps2}
    (junction 16) -> (junction 15) [order 1] : [DeltaSpeed <= MINUSONE_FLOAT * KVMC_SpdCtrlEnBand_kph && SpdCtrlFlag == 0]
    (junction 16) -> (junction 20) [order 2]
    (junction 15) -> (junction 12) : {SpdCtrlFlag = 1;
        |  ReqAccel = KVMC_SpdCtrlReqAccel_mps2}
    (junction 20) -> (junction 18) [order 1] : [SpdCtrlFlag == 1]
    (junction 18) -> (junction 24) [order 1] : [ReqAccel > ZERO_FLOAT]
    (junction 24) -> (junction 26) [order 1] : [DeltaSpeed >= KVMC_SpdCtrlDisBand_kph]
    (junction 20) -> (junction 42) [order 2] : {SpdCtrlFlag = 0}
    (junction 18) -> (junction 40) [order 2]
    (junction 24) -> (junction 30) [order 2] : {SpdCtrlFlag = 1;
        |  ReqAccel = KVMC_SpdCtrlReqAccel_mps2}
    (junction 26) -> (junction 28) : {SpdCtrlFlag = 0;
        |  ReqAccel = ZERO_FLOAT}
    (junction 40) -> (junction 37) [order 1] : [ReqAccel < ZERO_FLOAT]
    (junction 37) -> (junction 33) [order 1] : [DeltaSpeed <= MINUSONE_FLOAT * KVMC_SpdCtrlDisBand_kph]
    (junction 40) -> (junction 49) [order 2]
    (junction 37) -> (junction 35) [order 2] : {SpdCtrlFlag = 1;
        |  ReqAccel = MINUSONE_FLOAT * KVMC_SpdCtrlReqAccel_mps2}
    (junction 33) -> (junction 38) : {SpdCtrlFlag = 0;
        |  ReqAccel = ZERO_FLOAT}
  data: DeltaSpeed input single; SpdCtrlFlag local boolean; ReqAccel output single; KVMC_SpdCtrlEnBand_kph input single; KVMC_SpdCtrlDisBand_kph input single; MINUSONE_FLOAT input single; KVMC_SpdCtrlReqAccel_mps2 input single; ZERO_FLOAT input single

== stateflow chart vmc/VMC/VMC/Scheduler ==
  state Scheduler
    (default) -> (junction 3) : {counter = 0;}
    Scheduler -> (junction 3) : {counter++}
    (junction 3) -> (junction 5) [order 1] : [counter%%2 == 0]
    (junction 3) -> (junction 11) [order 2]
    (junction 5) -> (junction 7) : {Trigger_10ms_1;
        |  counter = 0;}
    (junction 7) -> (junction 11)
  data: counter local uint8
  events: Trigger_10ms_1 output FUNCTION_CALL_EVENT

== stateflow chart vmc/VMC/VMC/SafetyControl/LatAccRollingAverage/RollingAverage ==
  state LatAccelRollingAverage
    (default) -> (junction 2) : {VVMC_RollAveCount_enum = ONE_INT}
    LatAccelRollingAverage -> (junction 2)
    (junction 2) -> (junction 3) : {VVMC_LatAccRollAve_Gps = ZERO_FLOAT}
    (junction 3) -> (junction 100) [order 1] : [VVMC_RollAveCount_enum < KVMC_LatAccRollAveLevel_enum]
    (junction 3) -> (junction 37) [order 2]
    (junction 100) -> (junction 5) : {% Memory
        |  VVMC_Memory_raw32[VVMC_RollAveCount_enum] = VINP_LatAccel_Gps;
        |
        |  % Memory Shift Counter
        |  VVMC_ShiftCount_enum = ONE_INT}
    (junction 5) -> (junction 7) [order 2]
    (junction 5) -> (junction 6) [order 1] : [VVMC_ShiftCount_enum <= VVMC_RollAveCount_enum]
    (junction 7) -> (junction 8) : {% Rolling Average
        |  VVMC_LatAccRollAve_Gps = VVMC_LatAccRollAve_Gps / VVMC_RollAveCount_enum;
        |
        |  % Rolling Average Counter
        |  VVMC_RollAveCount_enum++}
    (junction 35) -> (junction 5) : {VVMC_ShiftCount_enum++}
    (junction 6) -> (junction 36) : {% Rolling Average Sum
        |  VVMC_LatAccRollAve_Gps = VVMC_LatAccRollAve_Gps + VVMC_Memory_raw32[VVMC_ShiftCount_enum];
        |  }
    (junction 36) -> (junction 35)
    (junction 37) -> (junction 76) [order 1] : [VVMC_RollAveCount_enum == KVMC_LatAccRollAveLevel_enum]
    (junction 76) -> (junction 47)
    (junction 37) -> (junction 60) [order 2]
    (junction 78) -> (junction 76)
    (junction 47) -> (junction 30) : {% Memory
        |  VVMC_Memory_raw32[VVMC_RollAveCount_enum] = VINP_LatAccel_Gps;
        |
        |  % Memory Shift Counter
        |  VVMC_ShiftCount_enum = ONE_INT;
        | }
    (junction 60) -> (junction 62) [order 1] : [VVMC_RollAveCount_enum > KVMC_LatAccRollAveLevel_enum]
    (junction 60) -> (junction 39) [order 2]
    (junction 62) -> (junction 66) : {VVMC_MemoryShiftCount_enum = ONE_INT}
    (junction 30) -> (junction 48) [order 2]
    (junction 30) -> (junction 22) [order 1] : [VVMC_ShiftCount_enum <= VVMC_RollAveCount_enum]
    (junction 48) -> (junction 45) : {% Rolling Average
        |  VVMC_LatAccRollAve_Gps = VVMC_LatAccRollAve_Gps / VVMC_RollAveCount_enum;
        |
        |  % Memory Shift Counter
        |  VVMC_ShiftCount_enum = ONE_INT}
    (junction 14) -> (junction 30) : {VVMC_ShiftCount_enum++}
    (junction 22) -> (junction 25) : {% Rolling Average Sum
        |  VVMC_LatAccRollAve_Gps = VVMC_LatAccRollAve_Gps + VVMC_Memory_raw32[VVMC_ShiftCount_enum]}
    (junction 66) -> (junction 82) [order 2]
    (junction 66) -> (junction 69) [order 1] : [VVMC_MemoryShiftCount_enum < VVMC_RollAveCount_enum]
    (junction 82) -> (junction 80) : {VVMC_RollAveCount_enum = KVMC_LatAccRollAveLevel_enum}
    (junction 73) -> (junction 66) : {VVMC_MemoryShiftCount_enum++}
    (junction 69) -> (junction 71) : {VVMC_Memory_raw32[VVMC_MemoryShiftCount_enum] =...
        |  VVMC_Memory_raw32[VVMC_RollAveCount_enum - KVMC_LatAccRollAveLevel_enum + VVMC_MemoryShiftCount_enum]}
    (junction 25) -> (junction 14)
    (junction 71) -> (junction 73)
    (junction 80) -> (junction 78)
    (junction 45) -> (junction 39) [order 2]
    (junction 45) -> (junction 15) [order 1] : [VVMC_ShiftCount_enum < VVMC_RollAveCount_enum]
    (junction 41) -> (junction 45) : { VVMC_ShiftCount_enum++}
    (junction 15) -> (junction 38) : {% Gy Memory Shift
        |  VVMC_Memory_raw32[VVMC_ShiftCount_enum] = VVMC_Memory_raw32[VVMC_ShiftCount_enum + ONE_INT]}
    (junction 38) -> (junction 41)
  data: KVMC_LatAccRollAveLevel_enum input uint8; VVMC_ShiftCount_enum local uint8; VVMC_RollAveCount_enum local uint8; VVMC_Memory_raw32 local single size=100; ZERO_FLOAT input single; ONE_INT input uint8; VVMC_LatAccRollAve_Gps output single; VINP_LatAccel_Gps input single; VVMC_MemoryShiftCount_enum local uint8

== stateflow chart vmc/VMC/VMC/FeatureSetSpeed/SpeedDetermination ==
  state SpeedDetermination
    (default) -> (junction 9) : {VVMC_FeatSetSpdFinal_raw32 = ZERO_FLOAT}
    SpeedDetermination -> (junction 9)
    (junction 9) -> (junction 14) [order 1] : [VVMC_APPSpdLimit_flg == ENUM_APPSPDLIMIT_ON]
    (junction 14) -> (junction 16) [order 1] : [VTQD_SpdCtrlSta_flg == ENUM_SCPCRLSTA_ON]
    (junction 9) -> (junction 22) [order 2]
    (junction 14) -> (junction 20) [order 2] : {VVMC_FeatSetSpdFinal_raw32 = VVMC_APPSpdLimit_kph}
    (junction 16) -> (junction 18) : {VVMC_FeatSetSpdFinal_raw32 =...
        |  min(VVMC_APPSpdLimit_kph, VTQD_SetSpd_kph)}
    (junction 22) -> (junction 24) [order 1] : [VTQD_SpdCtrlSta_flg == ENUM_SCPCRLSTA_ON]
    (junction 22) -> (junction 28) [order 2] : {VVMC_FeatSetSpdFinal_raw32 = ZERO_FLOAT}
    (junction 24) -> (junction 26) : {VVMC_FeatSetSpdFinal_raw32 = VTQD_SetSpd_kph}
  data: VVMC_APPSpdLimit_flg input boolean; VTQD_SpdCtrlSta_flg input boolean; VVMC_APPSpdLimit_kph input single; VTQD_SetSpd_kph input single; ENUM_SCPCRLSTA_ON input uint8; ENUM_APPSPDLIMIT_ON input uint8; VVMC_FeatSetSpdFinal_raw32 output single; ZERO_FLOAT input single

== stateflow chart vmc/VMC/VMC/IMU/IMU sensing result /RollingAverage1 ==
  state RollingAverage
    (default) -> (junction 2) : {VVMC_RollAveCount_enum = ONE_INT}
    RollingAverage -> (junction 2)
    (junction 2) -> (junction 3) : {VVMC_RollAve_raw32 = ZERO_FLOAT}
    (junction 3) -> (junction 100) [order 1] : [VVMC_RollAveCount_enum < KVMC_RollAveLevel_enum]
    (junction 3) -> (junction 37) [order 2]
    (junction 100) -> (junction 5) : {% Memory
        |  VVMC_Memory_raw32[VVMC_RollAveCount_enum] = VINP_INPData_raw32;
        |
        |  % Memory Shift Counter
        |  VVMC_ShiftCount_enum = ONE_INT}
    (junction 5) -> (junction 7) [order 2]
    (junction 5) -> (junction 6) [order 1] : [VVMC_ShiftCount_enum <= VVMC_RollAveCount_enum]
    (junction 7) -> (junction 8) : {% Rolling Average
        |  VVMC_RollAve_raw32 = VVMC_RollAve_raw32 / VVMC_RollAveCount_enum;
        |
        |  % Rolling Average Counter
        |  VVMC_RollAveCount_enum++}
    (junction 35) -> (junction 5) : {VVMC_ShiftCount_enum++}
    (junction 6) -> (junction 36) : {% Rolling Average Sum
        |  VVMC_RollAve_raw32 = VVMC_RollAve_raw32 + VVMC_Memory_raw32[VVMC_ShiftCount_enum];
        |  }
    (junction 36) -> (junction 35)
    (junction 37) -> (junction 76) [order 1] : [VVMC_RollAveCount_enum == KVMC_RollAveLevel_enum]
    (junction 76) -> (junction 47)
    (junction 37) -> (junction 60) [order 2]
    (junction 78) -> (junction 76)
    (junction 47) -> (junction 30) : {% Memory
        |  VVMC_Memory_raw32[VVMC_RollAveCount_enum] = VINP_INPData_raw32;
        |
        |  % Memory Shift Counter
        |  VVMC_ShiftCount_enum = ONE_INT;
        | }
    (junction 60) -> (junction 62) [order 1] : [VVMC_RollAveCount_enum > KVMC_RollAveLevel_enum]
    (junction 60) -> (junction 39) [order 2]
    (junction 62) -> (junction 66) : {VVMC_MemoryShiftCount_enum = ONE_INT}
    (junction 30) -> (junction 48) [order 2]
    (junction 30) -> (junction 22) [order 1] : [VVMC_ShiftCount_enum <= VVMC_RollAveCount_enum]
    (junction 48) -> (junction 45) : {% Rolling Average
        |  VVMC_RollAve_raw32 = VVMC_RollAve_raw32 / VVMC_RollAveCount_enum;
        |
        |  % Memory Shift Counter
        |  VVMC_ShiftCount_enum = ONE_INT}
    (junction 14) -> (junction 30) : {VVMC_ShiftCount_enum++}
    (junction 22) -> (junction 25) : {% Rolling Average Sum
        |  VVMC_RollAve_raw32 = VVMC_RollAve_raw32 + VVMC_Memory_raw32[VVMC_ShiftCount_enum]}
    (junction 66) -> (junction 82) [order 2]
    (junction 66) -> (junction 69) [order 1] : [VVMC_MemoryShiftCount_enum < VVMC_RollAveCount_enum]
    (junction 82) -> (junction 80) : {VVMC_RollAveCount_enum = KVMC_RollAveLevel_enum}
    (junction 73) -> (junction 66) : {VVMC_MemoryShiftCount_enum++}
    (junction 69) -> (junction 71) : {VVMC_Memory_raw32[VVMC_MemoryShiftCount_enum] =...
        |  VVMC_Memory_raw32[VVMC_RollAveCount_enum - KVMC_RollAveLevel_enum + VVMC_MemoryShiftCount_enum]}
    (junction 25) -> (junction 14)
    (junction 71) -> (junction 73)
    (junction 80) -> (junction 78)
    (junction 45) -> (junction 39) [order 2]
    (junction 45) -> (junction 15) [order 1] : [VVMC_ShiftCount_enum < VVMC_RollAveCount_enum]
    (junction 41) -> (junction 45) : { VVMC_ShiftCount_enum++}
    (junction 15) -> (junction 38) : {% Gy Memory Shift
        |  VVMC_Memory_raw32[VVMC_ShiftCount_enum] = VVMC_Memory_raw32[VVMC_ShiftCount_enum + ONE_INT]}
    (junction 38) -> (junction 41)
  data: KVMC_RollAveLevel_enum input uint8; VVMC_ShiftCount_enum local uint8; VVMC_RollAveCount_enum local uint8; VVMC_Memory_raw32 local single size=100; ZERO_FLOAT input single; ONE_INT input uint8; VVMC_RollAve_raw32 output single; VINP_INPData_raw32 input single; VVMC_MemoryShiftCount_enum local uint8

== stateflow chart vmc/VMC/VMC/SafetyControl/LKAStrgTqRollingAverage ==
  state LKAStrgTqRollingAverage
    (default) -> (junction 2) : {VVMC_RollAveCount_enum = ONE_INT}
    LKAStrgTqRollingAverage -> (junction 2)
    (junction 2) -> (junction 3) : {VVMC_LKAStrgTqRollAve_Nm = ZERO_FLOAT}
    (junction 3) -> (junction 100) [order 1] : [VVMC_RollAveCount_enum < KVMC_LKAStrgTqRollAveLevel_enum]
    (junction 3) -> (junction 37) [order 2]
    (junction 100) -> (junction 5) : {% Memory
        |  VVMC_LKAStrgTqMemory_Nm[VVMC_RollAveCount_enum] = VINP_LKAStrToqReq_Nm;
        |
        |  % Memory Shift Counter
        |  VVMC_LKAStrgTqShiftCount_enum = ONE_INT}
    (junction 5) -> (junction 7) [order 2]
    (junction 5) -> (junction 6) [order 1] : [VVMC_LKAStrgTqShiftCount_enum <= VVMC_RollAveCount_enum]
    (junction 7) -> (junction 8) : {% Rolling Average
        |  VVMC_LKAStrgTqRollAve_Nm = VVMC_LKAStrgTqRollAve_Nm / VVMC_RollAveCount_enum;
        |
        |  % Rolling Average Counter
        |  VVMC_RollAveCount_enum++}
    (junction 35) -> (junction 5) : {VVMC_LKAStrgTqShiftCount_enum++}
    (junction 6) -> (junction 36) : {% Rolling Average Sum
        |  VVMC_LKAStrgTqRollAve_Nm = VVMC_LKAStrgTqRollAve_Nm + VVMC_LKAStrgTqMemory_Nm[VVMC_LKAStrgTqShiftCount_enum];
        |  }
    (junction 36) -> (junction 35)
    (junction 37) -> (junction 76) [order 1] : [VVMC_RollAveCount_enum == KVMC_LKAStrgTqRollAveLevel_enum]
    (junction 76) -> (junction 47)
    (junction 37) -> (junction 60) [order 2]
    (junction 78) -> (junction 76)
    (junction 47) -> (junction 30) : {% Memory
        |  VVMC_LKAStrgTqMemory_Nm[VVMC_RollAveCount_enum] = VINP_LKAStrToqReq_Nm;
        |
        |  % Memory Shift Counter
        |  VVMC_LKAStrgTqShiftCount_enum = ONE_INT;
        | }
    (junction 60) -> (junction 62) [order 1] : [VVMC_RollAveCount_enum > KVMC_LKAStrgTqRollAveLevel_enum]
    (junction 60) -> (junction 39) [order 2]
    (junction 62) -> (junction 66) : {VVMC_MemoryShiftCount_enum = ONE_INT}
    (junction 30) -> (junction 48) [order 2]
    (junction 30) -> (junction 22) [order 1] : [VVMC_LKAStrgTqShiftCount_enum <= VVMC_RollAveCount_enum]
    (junction 48) -> (junction 45) : {% Rolling Average
        |  VVMC_LKAStrgTqRollAve_Nm = VVMC_LKAStrgTqRollAve_Nm / VVMC_RollAveCount_enum;
        |
        |  % Memory Shift Counter
        |  VVMC_LKAStrgTqShiftCount_enum = ONE_INT}
    (junction 14) -> (junction 30) : {VVMC_LKAStrgTqShiftCount_enum++}
    (junction 22) -> (junction 25) : {% Rolling Average Sum
        |  VVMC_LKAStrgTqRollAve_Nm = VVMC_LKAStrgTqRollAve_Nm + VVMC_LKAStrgTqMemory_Nm[VVMC_LKAStrgTqShiftCount_enum]}
    (junction 66) -> (junction 82) [order 2]
    (junction 66) -> (junction 69) [order 1] : [VVMC_MemoryShiftCount_enum < VVMC_RollAveCount_enum]
    (junction 82) -> (junction 80) : {VVMC_RollAveCount_enum = KVMC_LKAStrgTqRollAveLevel_enum}
    (junction 73) -> (junction 66) : {VVMC_MemoryShiftCount_enum++}
    (junction 69) -> (junction 71) : {VVMC_LKAStrgTqMemory_Nm[VVMC_MemoryShiftCount_enum] =...
        |  VVMC_LKAStrgTqMemory_Nm[VVMC_RollAveCount_enum - KVMC_LKAStrgTqRollAveLevel_enum + VVMC_MemoryShiftCount_enum]}
    (junction 25) -> (junction 14)
    (junction 71) -> (junction 73)
    (junction 80) -> (junction 78)
    (junction 45) -> (junction 39) [order 2]
    (junction 45) -> (junction 15) [order 1] : [VVMC_LKAStrgTqShiftCount_enum < VVMC_RollAveCount_enum]
    (junction 41) -> (junction 45) : { VVMC_LKAStrgTqShiftCount_enum++}
    (junction 15) -> (junction 38) : {% Gy Memory Shift
        |  VVMC_LKAStrgTqMemory_Nm[VVMC_LKAStrgTqShiftCount_enum] = VVMC_LKAStrgTqMemory_Nm[VVMC_LKAStrgTqShiftCount_enum + ONE_INT]}
    (junction 38) -> (junction 41)
  data: KVMC_LKAStrgTqRollAveLevel_enum input uint8; VVMC_LKAStrgTqShiftCount_enum local uint8; VVMC_RollAveCount_enum local uint8; VVMC_LKAStrgTqMemory_Nm local single size=100; ZERO_FLOAT input single; ONE_INT input uint8; VVMC_LKAStrgTqRollAve_Nm output single; VINP_LKAStrToqReq_Nm input single; VVMC_MemoryShiftCount_enum local uint8
